simulink model "flightPitchControl"  (R2022a)
settings: Solver=VariableStepAuto  StartTime=0.0  StopTime=500  RelTol=1e-3
libraries: cstblocks x2, simulink_extras x1
settings Model: Creator=noahcurran  LastModifiedBy=noahcurran

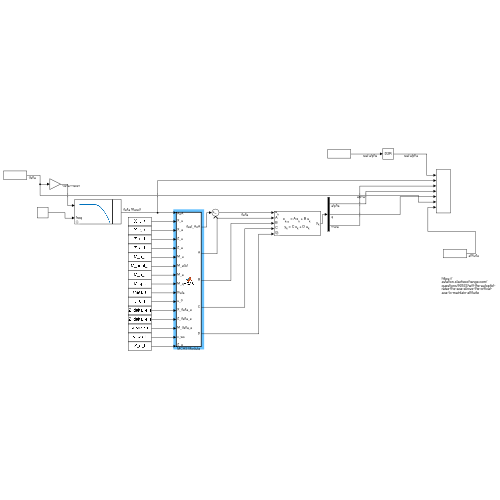
[thumbnail: Simulink's stored preview of the top-level diagram]
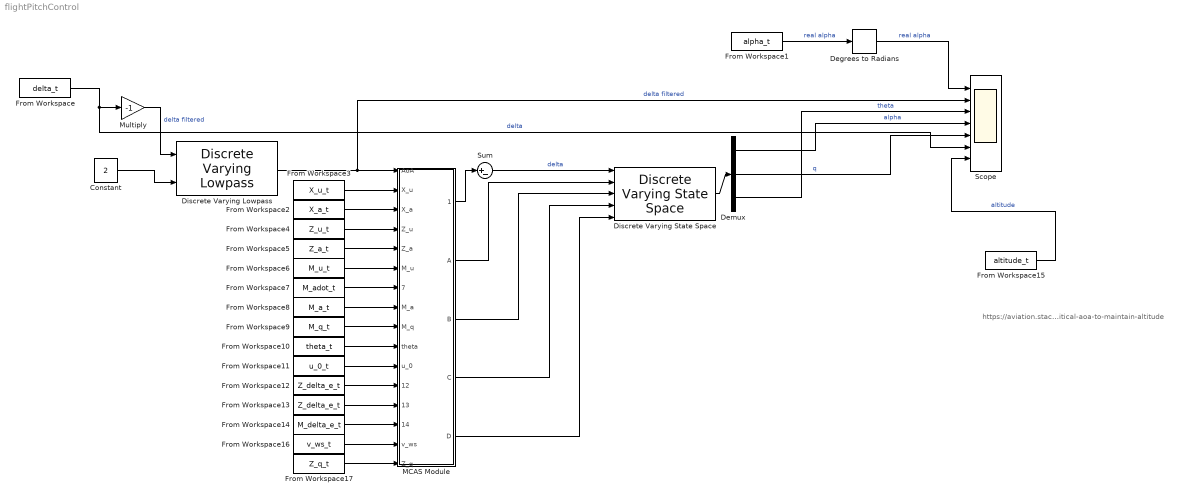
== system flightPitchControl ==
  note: https://aviation.stackexchange.com/questions/92522/will-the-autopilot-raise-the-aoa-above-the-critical-aoa-to-maintain-altitude
  Constant : Constant  Value=2
  Degrees to Radians : simulink_extras/Transformations/Degrees to Radians
  Demux : Demux  Outputs=3
  Discrete Varying Lowpass : cstblocks/Linear Parameter Varying/Discrete Varying Lowpass  N=7  w0=0  Ts=0.1
      settings: SourceProductBaseCode=CT
  Discrete Varying State Space : cstblocks/Linear Parameter Varying/Discrete Varying State Space  x0=0  Ts=-1  OutputX=off  OutputDX=off
      settings: SourceProductBaseCode=CT
  From Workspace : FromWorkspace  VariableName=delta_t  OutDataTypeStr=double  SampleTime=0.1  Interpolate=off  OutputAfterFinalValue=Setting to zero
  From Workspace1 : FromWorkspace  VariableName=alpha_t  SampleTime=0.1  Interpolate=off  OutputAfterFinalValue=Setting to zero
  From Workspace10 : FromWorkspace  VariableName=theta_t  OutDataTypeStr=double  SampleTime=0.1  Interpolate=off  OutputAfterFinalValue=Setting to zero
  From Workspace11 : FromWorkspace  VariableName=u_0_t  OutDataTypeStr=double  SampleTime=0.1  Interpolate=off  OutputAfterFinalValue=Setting to zero
  From Workspace12 : FromWorkspace  VariableName=Z_delta_e_t  OutDataTypeStr=double  SampleTime=0.1  Interpolate=off  OutputAfterFinalValue=Setting to zero
  From Workspace13 : FromWorkspace  VariableName=Z_delta_e_t  OutDataTypeStr=double  SampleTime=0.1  Interpolate=off  OutputAfterFinalValue=Setting to zero
  From Workspace14 : FromWorkspace  VariableName=M_delta_e_t  OutDataTypeStr=double  SampleTime=0.1  Interpolate=off  OutputAfterFinalValue=Setting to zero
  From Workspace15 : FromWorkspace  VariableName=altitude_t  SampleTime=0.1  Interpolate=off  OutputAfterFinalValue=Setting to zero
  From Workspace16 : FromWorkspace  VariableName=v_ws_t  OutDataTypeStr=double  SampleTime=0.1  Interpolate=off  OutputAfterFinalValue=Setting to zero
  From Workspace17 : FromWorkspace  VariableName=Z_q_t  OutDataTypeStr=double  SampleTime=0.1  Interpolate=off  OutputAfterFinalValue=Setting to zero
  From Workspace2 : FromWorkspace  VariableName=X_a_t  OutDataTypeStr=double  SampleTime=0.1  Interpolate=off  OutputAfterFinalValue=Setting to zero
  From Workspace3 : FromWorkspace  VariableName=X_u_t  OutDataTypeStr=double  SampleTime=0.1  Interpolate=off  OutputAfterFinalValue=Setting to zero
  From Workspace4 : FromWorkspace  VariableName=Z_u_t  OutDataTypeStr=double  SampleTime=0.1  Interpolate=off  OutputAfterFinalValue=Setting to zero
  From Workspace5 : FromWorkspace  VariableName=Z_a_t  OutDataTypeStr=double  SampleTime=0.1  Interpolate=off  OutputAfterFinalValue=Setting to zero
  From Workspace6 : FromWorkspace  VariableName=M_u_t  OutDataTypeStr=double  SampleTime=0.1  Interpolate=off  OutputAfterFinalValue=Setting to zero
  From Workspace7 : FromWorkspace  VariableName=M_adot_t  OutDataTypeStr=double  SampleTime=0.1  Interpolate=off  OutputAfterFinalValue=Setting to zero
  From Workspace8 : FromWorkspace  VariableName=M_a_t  OutDataTypeStr=double  SampleTime=0.1  Interpolate=off  OutputAfterFinalValue=Setting to zero
  From Workspace9 : FromWorkspace  VariableName=M_q_t  OutDataTypeStr=double  SampleTime=0.1  Interpolate=off  OutputAfterFinalValue=Setting to zero
  MCAS Module : MATLAB Function  TreatAsAtomicUnit=on
  Multiply : Gain  Gain=-1
  Scope : Scope  NumInputPorts=7
  Sum : Sum  Inputs=|+-
  wires:
  Demux/1 -> Scope/4  "alpha"
  Sum/1 -> Discrete Varying State Space/1  "delta"
  MCAS Module/1(dest_AoA) -> Sum/1
  From Workspace/1 -> Scope/6, Multiply/1  "delta"
  From Workspace1/1 -> Degrees to Radians/1  "real alpha"
  From Workspace3/1 -> MCAS Module/2(X_u)
  From Workspace2/1 -> MCAS Module/3(X_a)
  From Workspace11/1 -> MCAS Module/11(u_0)
  From Workspace4/1 -> MCAS Module/4(Z_u)
  From Workspace5/1 -> MCAS Module/5(Z_a)
  From Workspace6/1 -> MCAS Module/6(M_u)
  From Workspace7/1 -> MCAS Module/7(M_adot)
  From Workspace8/1 -> MCAS Module/8(M_a)
  From Workspace9/1 -> MCAS Module/9(M_q)
  From Workspace12/1 -> MCAS Module/12(X_delta_e)
  From Workspace13/1 -> MCAS Module/13(Z_delta_e)
  From Workspace14/1 -> MCAS Module/14(M_delta_e)
  Discrete Varying State Space/1 -> Demux/1
  MCAS Module/2(A) -> Discrete Varying State Space/2
  MCAS Module/3(B) -> Discrete Varying State Space/3
  MCAS Module/4(C) -> Discrete Varying State Space/4
  MCAS Module/5(D) -> Discrete Varying State Space/5
  Demux/2 -> Scope/5  "q"
  Demux/3 -> Scope/3  "theta"
  Degrees to Radians/1 -> Scope/1  "real alpha"
  Discrete Varying Lowpass/1 -> MCAS Module/1(AoA), Scope/2  "delta filtered"
  Constant/1 -> Discrete Varying Lowpass/2
  From Workspace15/1 -> Scope/7  "altitude"
  Multiply/1 -> Discrete Varying Lowpass/1  "delta filtered"
  From Workspace10/1 -> MCAS Module/10(theta)
  From Workspace16/1 -> MCAS Module/15(v_ws)
  From Workspace17/1 -> MCAS Module/16(Z_q)

== matlab function flightPitchControl/MCAS Module ==
  data: AoA input; dest_AoA output; X_u input; X_a input; Z_u input; Z_a input; M_u input; M_adot input; M_a input; M_q input; theta input; u_0 input; X_delta_e input; Z_delta_e input; M_delta_e input; A output; B output; C output; D output; v_ws input; Z_q input
function [dest_AoA, A, B, C, D] = MCAS(AoA, X_u, X_a, Z_u, Z_a, M_u, M_adot, M_a, M_q, theta, u_0, X_delta_e, Z_delta_e, M_delta_e, v_ws, Z_q)
    g = 32.2; %(gravity), ft/s^2
    
    dest_AoA = AoA;
    
    % http://article.sapub.org/image/10.5923.j.jmea.20130301.02_001.gif

    A = [
                Z_a/v_ws        (v_ws + Z_q)/v_ws   0;%-g*sin(theta)/v_ws;
                M_a             M_q                 0;
                0               1                   0;
        ];
    
        
    B = [
                Z_delta_e/v_ws;
                M_delta_e;
                0;
        ];

    C = eye(3);
    D = [0; 0; 0];
end
